simulink library "Vb_Converter_lib"  (Simulink 7.2)
settings: Solver=ode45  SolverMode=SingleTasking  StartTime=0.0  StopTime=10.0  RelTol=1e-3
libraries: simulink x2
settings Model: Creator=cbuttril  LastModifiedBy=mahill

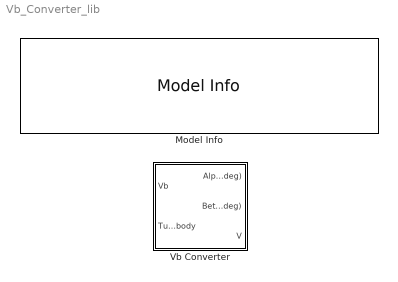
== system Vb_Converter_lib ==
  Model Info : simulink/Model-Wide Utilities/Model Info  SystemSampleTime=-1  InitialBlockCM=None  BlockCM=None  Frame=on  DisplayStringWithTags=|  HorizontalTextAlignment=Center  LeftAlignmentValue=0.5  SourceBlockDiagram=Vb_Converter_lib  TagMaxNumber=20
      | Developed using Matlab Release 2007a
      | 
      | SVN:%<ModelVersion>
      | Last modifed by %<LastModifiedBy> on %<LastModificationDate>
  Vb Converter : Subsystem

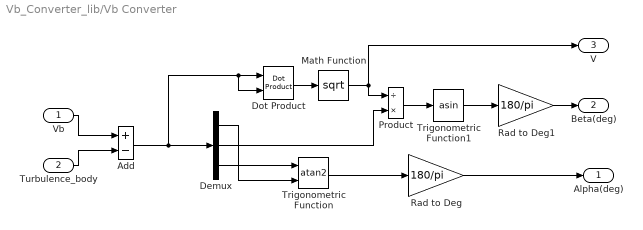
== system Vb_Converter_lib/Vb Converter ==
  Vb : Inport  OutDataType=sfix(16)  OutScaling=2^0
  Turbulence_body : Inport  Port=2  OutDataType=sfix(16)  OutScaling=2^0
  Add : Sum  Inputs=+-  OutDataType=sfix(16)  OutScaling=2^-10
  Demux : Demux  Outputs=3
  Dot Product : simulink/Math Operations/Dot Product  InputSameDT=on  OutDataType=sfix(16)  OutScaling=2^-10  DoSatur=off
  Math Function : Math  Operator=sqrt  OutDataType=sfix(16)  OutScaling=2^0  SaturateOnIntegerOverflow=on
  Product : Product  Inputs=/*  OutDataType=sfix(16)  OutScaling=2^0  SaturateOnIntegerOverflow=on  OutDataTypeStr=Inherit: Same as first input
  Rad to Deg : Gain  Gain=180/pi  ParameterDataType=sfix(16)  ParameterScaling=2^0  OutDataType=sfix(16)  OutScaling=2^0  SaturateOnIntegerOverflow=on  OutDataTypeStr=Inherit: Same as input  ParamDataTypeStr=Inherit: Same as input
  Rad to Deg1 : Gain  Gain=180/pi  ParameterDataType=sfix(16)  ParameterScaling=2^0  OutDataType=sfix(16)  OutScaling=2^0  SaturateOnIntegerOverflow=on  OutDataTypeStr=Inherit: Same as input  ParamDataTypeStr=Inherit: Same as input
  Trigonometric Function : Trigonometry  Operator=atan2
  Trigonometric Function1 : Trigonometry  Operator=asin
  Alpha(deg) : Outport  OutDataType=sfix(16)  OutScaling=2^0
  Beta(deg) : Outport  Port=2  OutDataType=sfix(16)  OutScaling=2^0
  V : Outport  Port=3  OutDataType=sfix(16)  OutScaling=2^0
  wires:
  Rad to Deg1/1 -> Beta(deg)/1
  Trigonometric Function1/1 -> Rad to Deg1/1
  Rad to Deg/1 -> Alpha(deg)/1
  Trigonometric Function/1 -> Rad to Deg/1
  Dot Product/1 -> Math Function/1
  Demux/1 -> Trigonometric Function/2
  Demux/3 -> Trigonometric Function/1
  Product/1 -> Trigonometric Function1/1
  Math Function/1 -> Product/1, V/1
  Demux/2 -> Product/2
  Turbulence_body/1 -> Add/2
  Vb/1 -> Add/1
  Add/1 -> Demux/1, Dot Product/1, Dot Product/2
